simulink model "HVDCMMCInterconnection_O"  (R2023b)
settings: Solver=FixedStepDiscrete  StartTime=0.0  StopTime=10  RelTol=1e-3  EnableMultiTasking=on
PreLoadFcn:
  | HVDCMMCInterconnectionParam
StartFcn:
  | tic
StopFcn:
  | toc
values from neighbouring files (symbols this model uses):
  C_PM = 1.758e-3    (= 0.001758)    [HVDCMMCInterconnectionParam.m]
  Cfilter = 1/(Larm*wc2)    (= 4.78421193241e-05)    [HVDCMMCInterconnectionParam.m]
  Cg = 50e-9    (= 5e-08)    [HVDCMMCInterconnectionParam.m]
  Fc = Fnom*3.37    (= 168.5)    [HVDCMMCInterconnectionParam.m]
  Fnom = 50    [HVDCMMCInterconnectionParam.m]
  Ki_Ireg = 6    [HVDCMMCInterconnectionParam.m]
  Ki_Preg = 1.0    (= 1)    [HVDCMMCInterconnectionParam.m]
  Ki_Qreg = 1.0    (= 1)    [HVDCMMCInterconnectionParam.m]
  Ki_VDCreg = 100    [HVDCMMCInterconnectionParam.m]
  Kp_Ireg = 0.6    [HVDCMMCInterconnectionParam.m]
  Kp_Preg = 0.5/3    (= 0.166666666667)    [HVDCMMCInterconnectionParam.m]
  Kp_Qreg = 0.5/3    (= 0.166666666667)    [HVDCMMCInterconnectionParam.m]
  Kp_VDCreg = 4    [HVDCMMCInterconnectionParam.m]
  L_cable = 15e-3    (= 0.015)    [HVDCMMCInterconnectionParam.m]
  Larm = Larm_pu*(Zbase/(2*pi*Fnom))    (= 0.0529455974536)    [HVDCMMCInterconnectionParam.m]
  Lff = Larm_pu/2    (= 0.075)    [HVDCMMCInterconnectionParam.m]
  Limits_Ireg = [ 2.0  -2.0]    [HVDCMMCInterconnectionParam.m]
  Limits_Preg = [ 1.2, 0.8 ]    [HVDCMMCInterconnectionParam.m]
  Limits_Qreg = [ 0.25, -0.25 ]    [HVDCMMCInterconnectionParam.m]
  Limits_VDCreg = [ 2.0  -2.0]    [HVDCMMCInterconnectionParam.m]
  Lxfo = 0.12    [HVDCMMCInterconnectionParam.m]
  Nb_PM = 36    [HVDCMMCInterconnectionParam.m]
  Pnom = 1000e6    (= 1000000000)    [HVDCMMCInterconnectionParam.m]
  R_cable = 0.5    [HVDCMMCInterconnectionParam.m]
  R_startup = 400    [HVDCMMCInterconnectionParam.m]
  Rarm = Rarm_pu*Zbase    (= 0.1663335)    [HVDCMMCInterconnectionParam.m]
  Rff = Rarm_pu/2    (= 0.00075)    [HVDCMMCInterconnectionParam.m]
  Rfilter = 1/(Cfilter*w)*30    (= 1996.002)    [HVDCMMCInterconnectionParam.m]
  Rg = 100    [HVDCMMCInterconnectionParam.m]
  Rxfo = 0.003    [HVDCMMCInterconnectionParam.m]
  Slope_Pref = 0.5    [HVDCMMCInterconnectionParam.m]
  Slope_Qref = 0.5    [HVDCMMCInterconnectionParam.m]
  Slope_Vdc_ref = Vnom_dc/5    (= 128000)    [HVDCMMCInterconnectionParam.m]
  Tbrk1_On = 0.1    [HVDCMMCInterconnectionParam.m]
  Tbrk2_On = 1.0    (= 1)    [HVDCMMCInterconnectionParam.m]
  Tdeblock = 1.5    [HVDCMMCInterconnectionParam.m]
  Tfault = 9999    [HVDCMMCInterconnectionParam.m]
  Ton_Converter2 = 4    [HVDCMMCInterconnectionParam.m]
  Ton_PQreg = 4    [HVDCMMCInterconnectionParam.m]
  Ton_VDCreg = 1.5    [HVDCMMCInterconnectionParam.m]
  Ts = Ts_Control    (= 4e-05)    [HVDCMMCInterconnectionParam.m]
  Ts_Control = 40e-6    (= 4e-05)    [HVDCMMCInterconnectionParam.m]
  Ts_Power = 20e-6    (= 2e-05)    [HVDCMMCInterconnectionParam.m]
  Vnom_dc = 640e3    (= 640000)    [HVDCMMCInterconnectionParam.m]
  Vnom_prim = 400e3    (= 400000)    [HVDCMMCInterconnectionParam.m]
  Vnom_sec = 333e3    (= 333000)    [HVDCMMCInterconnectionParam.m]
undefined symbols (not defined in the file or in its folder): DiscIntNeverNeededParam, Pcc
libraries: spsSeriesRLCBranchLib x24, spsCurrentMeasurementLib x11, spsVoltageMeasurementLib x8, simulink x7, spsHalfBridgeMMCLib x6, powerlib_extras x3, spsIdealSwitchLib x3, spsBreakerLib x3, spsParallelRLCBranchLib x3, spsThreePhaseBreakerLib x2, spsMeanLib x2, spsSecondOrderFilterLib x2
(part 2 of 2)

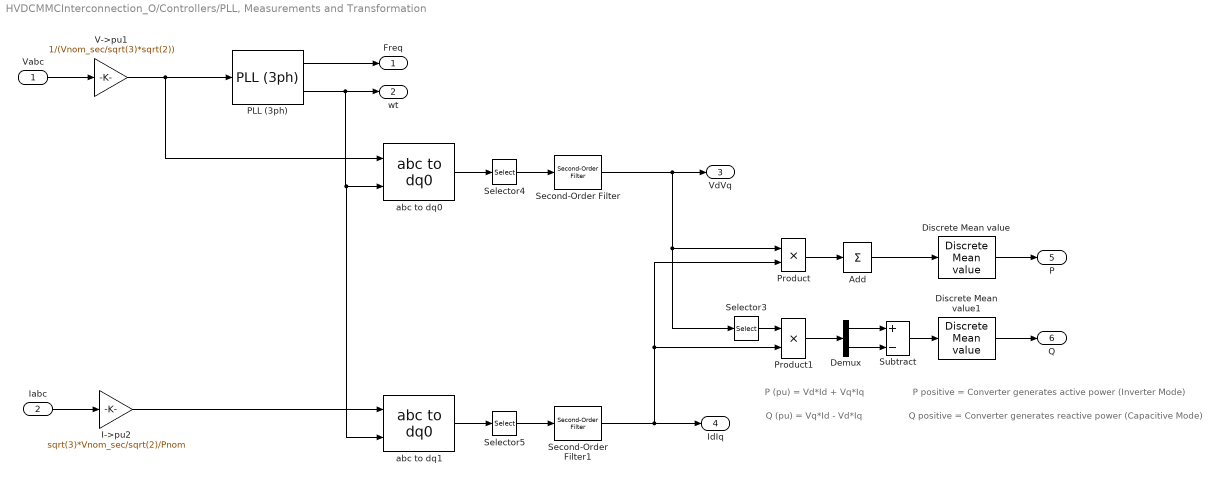
== system HVDCMMCInterconnection_O/Controllers/PLL, Measurements and Transformation ==
  note: P (pu) = Vd*Id + Vq*Iq
  note: Q (pu) = Vq*Id - Vd*Iq
  note: P positive = Converter generates active power (Inverter Mode)
  note: Q positive = Converter generates reactive power (Capacitive Mode)
  Vabc : Inport  PortDimensions=3
  Iabc : Inport  Port=2  PortDimensions=3
  Add : Sum  Inputs=1
  Demux : Demux  Outputs=2
  Discrete Mean value : powerlib_extras/Discrete Measurements/Discrete  Mean value  Freq=Fnom  Vinit=0  Ts=Ts
  Discrete Mean value1 : powerlib_extras/Discrete Measurements/Discrete  Mean value  Freq=Fnom  Vinit=0  Ts=Ts
  I->pu2 : Gain  Gain=sqrt(3)*Vnom_sec/sqrt(2)/Pnom  SaturateOnIntegerOverflow=on  OutDataTypeStr=Inherit: Same as input  ParamDataTypeStr=Inherit: Same as input
  PLL (3ph) : spsPLL3phLib/PLL (3ph)  Fmin=0.9*Fnom  Par_Init=[0, Fnom]  ParK=[180, 3200, 1]  TcD=1e-4  MaxRateChangeFreq=12  FilterCutOffFreq=25  Ts=Ts  AGC=on
  Product : Product  RndMeth=Zero
  Product1 : Product  RndMeth=Zero
  Second-Order Filter : spsSecondOrderFilterLib/Second-Order Filter  FilterType=Lowpass  Fo=Fn_filter  Zeta=Zeta_filter  Ts=Ts  Initialize=off  Vac_Init="[0,  0,  60]"  Vdc_Init=0  PlotResponse=off  FreqRange=[0, 500, 1]
  Second-Order Filter1 : spsSecondOrderFilterLib/Second-Order Filter  FilterType=Lowpass  Fo=Fn_filter  Zeta=Zeta_filter  Ts=Ts  Initialize=off  Vac_Init="[0,  0,  60]"  Vdc_Init=0  PlotResponse=off  FreqRange=[0, 500, 1]
  Selector3 : Selector  InputPortWidth=2  IndexOptions=Index vector (dialog)  Indices=[2 1]  OutputSizes=1
  Selector4 : Selector  InputPortWidth=3  IndexOptions=Index vector (dialog)  Indices=[1 2]  OutputSizes=1
  Selector5 : Selector  InputPortWidth=3  IndexOptions=Index vector (dialog)  Indices=[1 2]  OutputSizes=1
  Subtract : Sum  Inputs=+-
  V->pu1 : Gain  Gain=1/(Vnom_sec/sqrt(3)*sqrt(2))  SaturateOnIntegerOverflow=on  OutDataTypeStr=Inherit: Same as input  ParamDataTypeStr=Inherit: Same as input
  abc to dq0 : spsabctodq0Lib/abc to dq0  Alignment=90 degrees behind phase A axis
  abc to dq1 : spsabctodq0Lib/abc to dq0  Alignment=90 degrees behind phase A axis
  Freq : Outport
  wt : Outport  Port=2
  VdVq : Outport  Port=3
  IdIq : Outport  Port=4
  P : Outport  Port=5
  Q : Outport  Port=6
  wires:
  Selector3/1 -> Product1/1
  Discrete Mean value1/1 -> Q/1
  Discrete Mean value/1 -> P/1
  Second-Order Filter/1 -> VdVq/1, Product/1, Selector3/1
  Second-Order Filter1/1 -> IdIq/1, Product1/2, Product/2
  Product/1 -> Add/1
  Product1/1 -> Demux/1
  Demux/1 -> Subtract/1
  Demux/2 -> Subtract/2
  Add/1 -> Discrete Mean value/1
  Subtract/1 -> Discrete Mean value1/1
  abc to dq0/1 -> Selector4/1
  PLL (3ph)/1 -> Freq/1
  V->pu1/1 -> abc to dq0/1, PLL (3ph)/1
  Vabc/1 -> V->pu1/1
  PLL (3ph)/2 -> wt/1, abc to dq1/2, abc to dq0/2
  Iabc/1 -> I->pu2/1
  abc to dq1/1 -> Selector5/1
  I->pu2/1 -> abc to dq1/1
  Selector4/1 -> Second-Order Filter/1
  Selector5/1 -> Second-Order Filter1/1

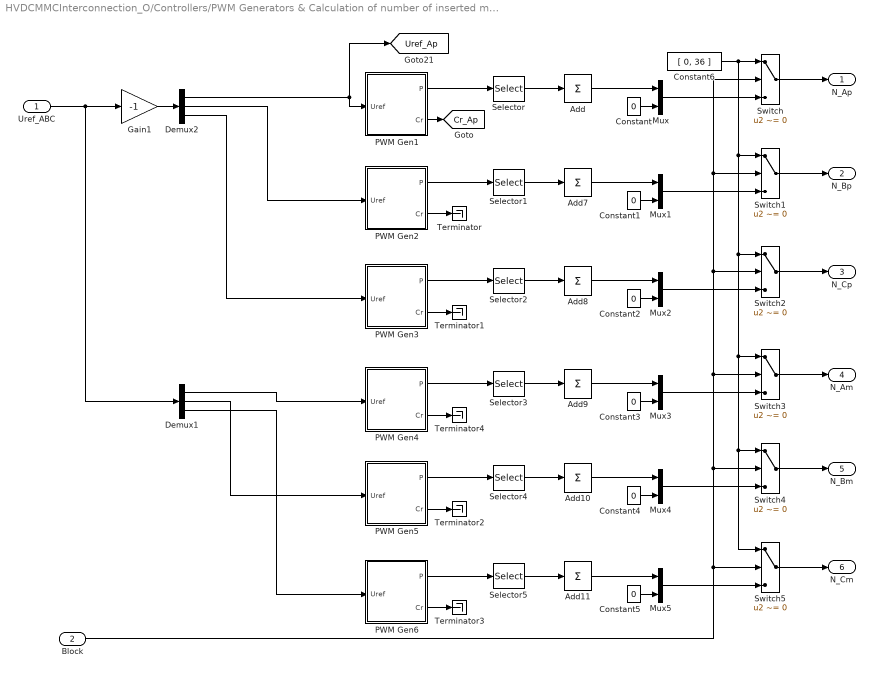
== system HVDCMMCInterconnection_O/Controllers/PWM Generators & Calculation of number of inserted modules (Nin) and number of blocked module (Nbl) ==
  Uref_ABC : Inport  PortDimensions=3
  Block : Inport  Port=2
  Add{,7..11} (6 alike) : Sum  Inputs=1
  Constant{,1..5} (6 alike) : Constant  Value=0
  Constant6 : Constant  Value=[ 0, 36 ]
  Demux1 : Demux  Outputs=3
  Demux2 : Demux  Outputs=3
  Gain1 : Gain  Gain=-1
  Mux{,1..5} (6 alike) : Mux  Inputs=2
  PWM Gen1 : Subsystem  mask(PWM generator for half-bridge MMC){n=Nb_PM, Fc=Fc, Ts=Ts_Power}
      mask prompts: n "Number of half-bridges"; Fc "Carriers frequency (Hz)"; Ts "Sample time (s)"
      mask init:
      | Tc=1/Fc;
      |         Pc= [ 0:360/n:360-360/n]*pi/180;
      |         Offset=Pc/(2*pi);
      |         Offset_Cr=Pc/(2*pi)*Tc;
      |         p=0;
      |         for m=1:2:2*n
      |             p=p+1;
      |             SelectPulsesPS(m)=p;
      |             SelectPulsesPS(m+1)=p+n;
      |         end
  PWM Gen2 : Subsystem  mask(PWM generator for half-bridge MMC){n=Nb_PM, Fc=Fc, Ts=Ts_Power}
      mask prompts: n "Number of half-bridges"; Fc "Carriers frequency (Hz)"; Ts "Sample time (s)"
      mask init: same as HVDCMMCInterconnection_O/Controllers/PWM Generators & Calculation of number of inserted modules (Nin) and number of blocked module (Nbl)/PWM Gen1
  PWM Gen3 : Subsystem  mask(PWM generator for half-bridge MMC){n=Nb_PM, Fc=Fc, Ts=Ts_Power}
      mask prompts: n "Number of half-bridges"; Fc "Carriers frequency (Hz)"; Ts "Sample time (s)"
      mask init: same as HVDCMMCInterconnection_O/Controllers/PWM Generators & Calculation of number of inserted modules (Nin) and number of blocked module (Nbl)/PWM Gen1
  PWM Gen4 : Subsystem  mask(PWM generator for half-bridge MMC){n=Nb_PM, Fc=Fc, Ts=Ts_Power}
      mask prompts: n "Number of half-bridges"; Fc "Carriers frequency (Hz)"; Ts "Sample time (s)"
      mask init: same as HVDCMMCInterconnection_O/Controllers/PWM Generators & Calculation of number of inserted modules (Nin) and number of blocked module (Nbl)/PWM Gen1
  PWM Gen5 : Subsystem  mask(PWM generator for half-bridge MMC){n=Nb_PM, Fc=Fc, Ts=Ts_Power}
      mask prompts: n "Number of half-bridges"; Fc "Carriers frequency (Hz)"; Ts "Sample time (s)"
      mask init: same as HVDCMMCInterconnection_O/Controllers/PWM Generators & Calculation of number of inserted modules (Nin) and number of blocked module (Nbl)/PWM Gen1
  PWM Gen6 : Subsystem  mask(PWM generator for half-bridge MMC){n=Nb_PM, Fc=Fc, Ts=Ts_Power}
      mask prompts: n "Number of half-bridges"; Fc "Carriers frequency (Hz)"; Ts "Sample time (s)"
      mask init: same as HVDCMMCInterconnection_O/Controllers/PWM Generators & Calculation of number of inserted modules (Nin) and number of blocked module (Nbl)/PWM Gen1
  Selector{,1..5} (6 alike) : Selector  InputPortWidth=72  IndexOptions=Index vector (dialog)  Indices=[1:2:71]  OutputSizes=1
  Switch{,1..5} (6 alike) : Switch  Criteria=u2 ~= 0  SaturateOnIntegerOverflow=off  InputSameDT=off
  Terminator{,1..4} (5 alike) : Terminator
  N_Ap : Outport
  N_Bp : Outport  Port=2
  N_Cp : Outport  Port=3
  N_Am : Outport  Port=4
  N_Bm : Outport  Port=5
  N_Cm : Outport  Port=6
  tag scope: Cr_Ap=global, Uref_Ap=global
  wires:
  PWM Gen4/2(Cr) -> Terminator4/1
  PWM Gen5/2(Cr) -> Terminator2/1
  Uref_ABC/1 -> Gain1/1, Demux1/1
  PWM Gen6/2(Cr) -> Terminator3/1
  PWM Gen2/2(Cr) -> Terminator/1
  Demux2/2 -> PWM Gen2/1(Uref)
  Demux2/1 -> PWM Gen1/1(Uref), [Uref_Ap]
  Gain1/1 -> Demux2/1
  PWM Gen1/2(Cr) -> [Cr_Ap]
  PWM Gen3/2(Cr) -> Terminator1/1
  Selector/1 -> Add/1
  Selector1/1 -> Add7/1
  Selector2/1 -> Add8/1
  Selector3/1 -> Add9/1
  Selector4/1 -> Add10/1
  Selector5/1 -> Add11/1
  Constant/1 -> Mux/2
  Add7/1 -> Mux1/1
  Constant1/1 -> Mux1/2
  Constant5/1 -> Mux5/2
  Switch/1 -> N_Ap/1
  Switch3/1 -> N_Am/1
  Mux1/1 -> Switch1/3
  Constant6/1 -> Switch/1, Switch5/1, Switch4/1, Switch3/1, Switch2/1, Switch1/1
  Constant2/1 -> Mux2/2
  Add9/1 -> Mux3/1
  Add8/1 -> Mux2/1
  Mux/1 -> Switch/3
  Switch1/1 -> N_Bp/1
  Constant4/1 -> Mux4/2
  Switch2/1 -> N_Cp/1
  Switch4/1 -> N_Bm/1
  Add/1 -> Mux/1
  Switch5/1 -> N_Cm/1
  Constant3/1 -> Mux3/2
  Add10/1 -> Mux4/1
  Add11/1 -> Mux5/1
  Block/1 -> Switch/2, Switch1/2, Switch2/2, Switch3/2, Switch4/2, Switch5/2
  Mux3/1 -> Switch3/3
  Mux4/1 -> Switch4/3
  Mux5/1 -> Switch5/3
  Mux2/1 -> Switch2/3
  PWM Gen6/1(P) -> Selector5/1
  PWM Gen5/1(P) -> Selector4/1
  PWM Gen4/1(P) -> Selector3/1
  PWM Gen3/1(P) -> Selector2/1
  PWM Gen2/1(P) -> Selector1/1
  PWM Gen1/1(P) -> Selector/1
  Demux2/3 -> PWM Gen3/1(Uref)
  Demux1/1 -> PWM Gen4/1(Uref)
  Demux1/3 -> PWM Gen6/1(Uref)
  Demux1/2 -> PWM Gen5/1(Uref)

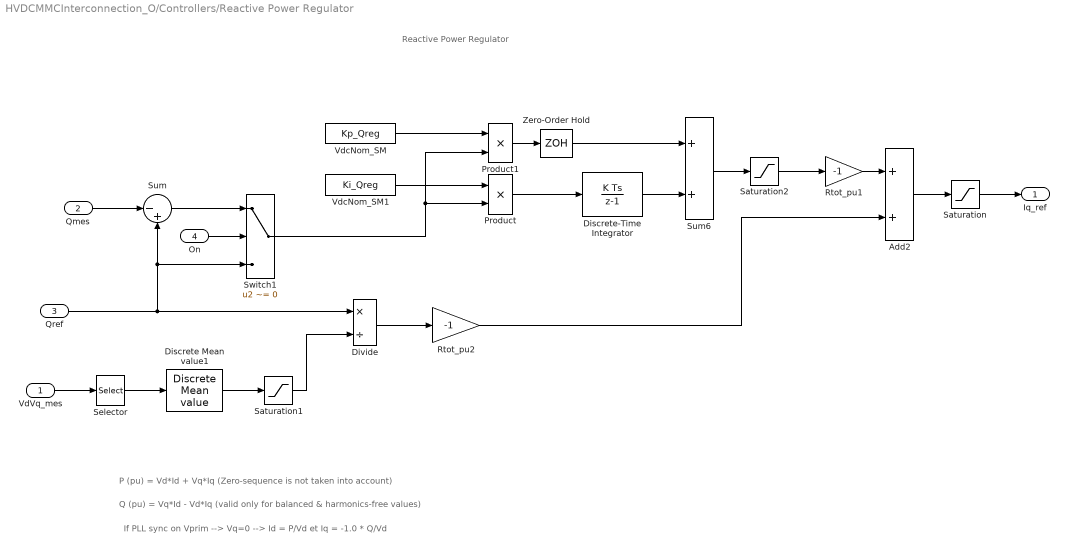
== system HVDCMMCInterconnection_O/Controllers/Reactive Power Regulator ==
  note: Reactive Power Regulator
  note: If PLL sync on Vprim --> Vq=0 --> Id = P/Vd et Iq = -1.0 * Q/Vd
  note: Q (pu) = Vq*Id - Vd*Iq (valid only for balanced & harmonics-free values)
  note: P (pu) = Vd*Id + Vq*Iq (Zero-sequence is not taken into account)
  VdVq_mes : Inport  PortDimensions=2
  Qmes : Inport  Port=2  PortDimensions=1
  Qref : Inport  Port=3  PortDimensions=1
  On : Inport  Port=4  PortDimensions=1
  Add2 : Sum
  Discrete Mean value1 : powerlib_extras/Discrete Measurements/Discrete  Mean value  Freq=Fnom  Vinit=0  Ts=Ts
  Discrete-Time Integrator : DiscreteIntegrator  SampleTime=Ts  LimitOutput=on  UpperSaturationLimit=Limits_Qreg(1)  LowerSaturationLimit=Limits_Qreg(2)  ICPrevOutput=DiscIntNeverNeededParam  ICPrevScaledInput=DiscIntNeverNeededParam
  Divide : Product  Inputs=*/
  Product : Product  RndMeth=Zero
  Product1 : Product  RndMeth=Zero
  Rtot_pu1 : Gain  Gain=-1  SaturateOnIntegerOverflow=on  OutDataTypeStr=Inherit: Same as input  ParamDataTypeStr=Inherit: Same as input
  Rtot_pu2 : Gain  Gain=-1  SaturateOnIntegerOverflow=on  OutDataTypeStr=Inherit: Same as input  ParamDataTypeStr=Inherit: Same as input
  Saturation : Saturate  UpperLimit=Limits_Qreg(1)  LowerLimit=Limits_Qreg(2)
  Saturation1 : Saturate  UpperLimit=2  LowerLimit=1e-6
  Saturation2 : Saturate  UpperLimit=Limits_Qreg(1)  LowerLimit=Limits_Qreg(2)
  Selector : Selector  InputPortWidth=2  IndexOptions=Index vector (dialog)  Indices=[1]  OutputSizes=1
  Sum : Sum  Inputs=|-+
  Sum6 : Sum  InputSameDT=on  SaturateOnIntegerOverflow=on  SampleTime=Ts  OutDataTypeStr=Inherit: Same as first input
  Switch1 : Switch  Criteria=u2 ~= 0  Threshold=0.5  OutDataTypeStr=double  SaturateOnIntegerOverflow=off  InputSameDT=off
  VdcNom_SM : Constant  Value=Kp_Qreg
  VdcNom_SM1 : Constant  Value=Ki_Qreg
  Zero-Order Hold : ZeroOrderHold  SampleTime=Ts
  Iq_ref : Outport
  wires:
  Saturation2/1 -> Rtot_pu1/1
  Saturation/1 -> Iq_ref/1
  Rtot_pu2/1 -> Add2/2
  Rtot_pu1/1 -> Add2/1
  Sum6/1 -> Saturation2/1
  Switch1/1 -> Product1/2, Product/2
  Sum/1 -> Switch1/1
  On/1 -> Switch1/2
  Add2/1 -> Saturation/1
  Product/1 -> Discrete-Time Integrator/1
  Product1/1 -> Zero-Order Hold/1
  VdcNom_SM/1 -> Product1/1
  VdcNom_SM1/1 -> Product/1
  Discrete-Time Integrator/1 -> Sum6/2
  Zero-Order Hold/1 -> Sum6/1
  Discrete Mean value1/1 -> Saturation1/1
  Saturation1/1 -> Divide/2
  Divide/1 -> Rtot_pu2/1
  Selector/1 -> Discrete Mean value1/1
  VdVq_mes/1 -> Selector/1
  Qmes/1 -> Sum/1
  Qref/1 -> Divide/1, Switch1/3, Sum/2

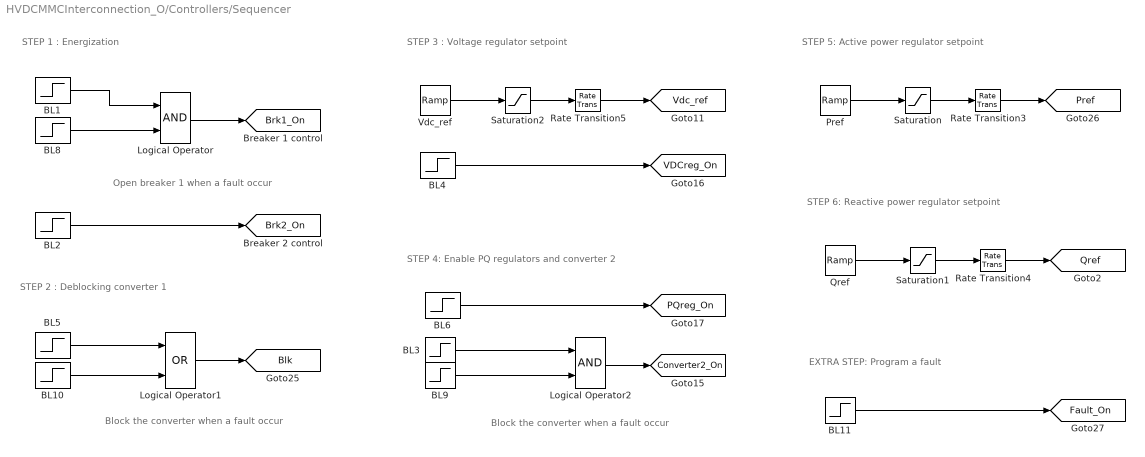
== system HVDCMMCInterconnection_O/Controllers/Sequencer ==
  note: Open breaker 1 when a fault occur
  note: Block the converter when a fault occur
  note: Block the converter when a fault occur
  note: STEP 6: Reactive power regulator setpoint
  note: STEP 4: Enable PQ regulators and converter 2
  note: STEP 5: Active power regulator setpoint
  note: STEP 3 : Voltage regulator setpoint
  note: STEP 2 : Deblocking converter 1
  note: STEP 1 : Energization
  note: EXTRA STEP: Program a fault
  BL1 : Step  Time=Tbrk1_On  SampleTime=Ts_Power
  BL10 : Step  Time=Tfault+Ts_Power  SampleTime=Ts_Power
  BL11 : Step  Time=Tfault  SampleTime=Ts_Power
  BL2 : Step  Time=Tbrk2_On  SampleTime=Ts_Power
  BL3 : Step  Time=Ton_Converter2  SampleTime=Ts_Power
  BL4 : Step  Time=Ton_VDCreg  SampleTime=Ts
  BL5 : Step  Time=Tdeblock  Before=1  After=0  SampleTime=Ts_Power
  BL6 : Step  Time=Ton_PQreg  SampleTime=Ts
  BL8 : Step  Time=Tfault + 1.95*(1/Fnom)  Before=1  After=0  SampleTime=Ts_Power
  BL9 : Step  Time=Tfault + 2*(1/Fnom)  Before=1  After=0  SampleTime=Ts_Power
  Logical Operator : Logic  AllPortsSameDT=off  OutDataTypeStr=boolean
  Logical Operator1 : Logic  Operator=OR  AllPortsSameDT=off  OutDataTypeStr=float('double')
  Logical Operator2 : Logic  AllPortsSameDT=off  OutDataTypeStr=boolean
  Pref : simulink/Sources/Ramp  slope=Slope_Pref  start=Tramping_Pref  InitialOutput=0
  Qref : simulink/Sources/Ramp  slope=Slope_Qref  start=Tramping_Qref  InitialOutput=0
  Rate Transition3 : RateTransition  OutPortSampleTime=Ts_Control
  Rate Transition4 : RateTransition  OutPortSampleTime=Ts_Control
  Rate Transition5 : RateTransition  OutPortSampleTime=Ts_Control
  Saturation : Saturate  UpperLimit=1  LowerLimit=-1
  Saturation1 : Saturate  UpperLimit=Limits_Qreg(1)  LowerLimit=Limits_Qreg(2)
  Saturation2 : Saturate  UpperLimit=Vnom_dc  LowerLimit=eps
  "Vdc_ref " : simulink/Sources/Ramp  slope=Slope_Vdc_ref  start=Tramping_Vdc_ref  InitialOutput=Vnom_sec*1.37
  tag scope: Blk=global, Brk1_On=global, Brk2_On=global, Converter2_On=global, Fault_On=global, PQreg_On=global, Pref=global, Qref=global, VDCreg_On=global, Vdc_ref=global
  wires:
  Saturation2/1 -> Rate Transition5/1
  Saturation1/1 -> Rate Transition4/1
  Pref/1 -> Saturation/1
  Qref/1 -> Saturation1/1
  Saturation/1 -> Rate Transition3/1
  Rate Transition3/1 -> [Pref]
  Rate Transition4/1 -> [Qref]
  Rate Transition5/1 -> [Vdc_ref]
  BL4/1 -> [VDCreg_On]
  BL6/1 -> [PQreg_On]
  "Vdc_ref "/1 -> Saturation2/1
  BL2/1 -> [Brk2_On]
  BL8/1 -> Logical Operator/2
  Logical Operator/1 -> [Brk1_On]
  BL1/1 -> Logical Operator/1
  BL9/1 -> Logical Operator2/2
  BL3/1 -> Logical Operator2/1
  Logical Operator2/1 -> [Converter2_On]
  Logical Operator1/1 -> [Blk]
  BL5/1 -> Logical Operator1/1
  BL10/1 -> Logical Operator1/2
  BL11/1 -> [Fault_On]

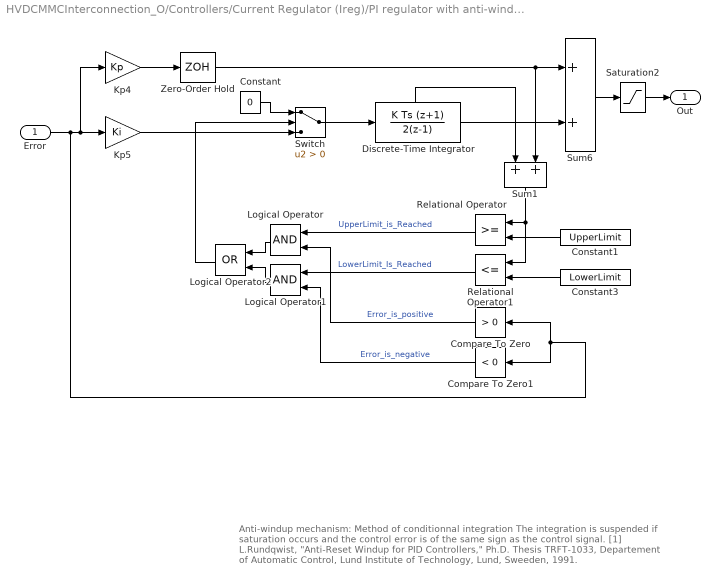
== system HVDCMMCInterconnection_O/Controllers/Current Regulator (Ireg)/PI regulator with anti-windup D ==
  note: Anti-windup mechanism: Method of conditionnal integration
      |
      | The integration is suspended if saturation occurs and the
      | control error is of the same sign as the control signal.
      |
      | [1] L.Rundqwist, "Anti-Reset Windup for PID Controllers," Ph.D. Thesis TRFT-1033,
      | Departement of Automatic Control, Lund Institute of Technology, Lund, Sweeden, 1991.
  Error : Inport  SampleTime=Ts
  Compare To Zero : simulink/Logic and Bit Operations/Compare To Zero  relop=>  OutDataTypeStr=uint8  ZeroCross=off
  Compare To Zero1 : simulink/Logic and Bit Operations/Compare To Zero  relop=<  OutDataTypeStr=uint8  ZeroCross=off
  Constant : Constant  Value=0
  Constant1 : Constant  Value=UpperLimit
  Constant3 : Constant  Value=LowerLimit
  Discrete-Time Integrator : DiscreteIntegrator  IntegratorMethod=Integration: Trapezoidal  InitialCondition=Init  SampleTime=Ts  LimitOutput=on  UpperSaturationLimit=UpperLimit  LowerSaturationLimit=LowerLimit  ShowStatePort=on  ICPrevOutput=DiscIntNeverNeededParam  ICPrevScaledInput=DiscIntNeverNeededParam
  Kp4 : Gain  Gain=Kp  SaturateOnIntegerOverflow=on  SampleTime=Ts  OutDataTypeStr=Inherit: Same as input  ParamDataTypeStr=Inherit: Same as input
  Kp5 : Gain  Gain=Ki  SaturateOnIntegerOverflow=on  SampleTime=Ts  OutDataTypeStr=Inherit: Same as input  ParamDataTypeStr=Inherit: Same as input
  Logical Operator : Logic  AllPortsSameDT=off  OutDataTypeStr=boolean
  Logical Operator1 : Logic  AllPortsSameDT=off  OutDataTypeStr=boolean
  Logical Operator2 : Logic  Operator=OR  AllPortsSameDT=off  OutDataTypeStr=boolean
  Relational Operator : RelationalOperator  OutDataTypeStr=boolean  InputSameDT=off
  Relational Operator1 : RelationalOperator  Operator=<=  OutDataTypeStr=boolean  InputSameDT=off
  Saturation2 : Saturate  UpperLimit=UpperLimit  LowerLimit=LowerLimit  SampleTime=Ts
  Sum1 : Sum  InputSameDT=on  SaturateOnIntegerOverflow=on  SampleTime=Ts  OutDataTypeStr=Inherit: Same as first input
  Sum6 : Sum  InputSameDT=on  SaturateOnIntegerOverflow=on  SampleTime=Ts  OutDataTypeStr=Inherit: Same as first input
  Switch : Switch  Criteria=u2 > Threshold  SaturateOnIntegerOverflow=off  InputSameDT=off
  Zero-Order Hold : ZeroOrderHold  SampleTime=Ts
  Out : Outport  SampleTime=Ts  InitialOutput=0
  wires:
  Constant/1 -> Switch/1
  Zero-Order Hold/1 -> Sum1/2, Sum6/1
  Discrete-Time Integrator/State -> Sum1/1
  Sum1/1 -> Relational Operator1/1, Relational Operator/1
  Logical Operator2/1 -> Switch/2
  Relational Operator/1 -> Logical Operator/1  "UpperLimit_is_Reached"
  Relational Operator1/1 -> Logical Operator1/1  "LowerLimit_Is_Reached"
  Constant1/1 -> Relational Operator/2
  Constant3/1 -> Relational Operator1/2
  Compare To Zero/1 -> Logical Operator/2  "Error_is_positive"
  Logical Operator/1 -> Logical Operator2/1
  Logical Operator1/1 -> Logical Operator2/2
  Compare To Zero1/1 -> Logical Operator1/2  "Error_is_negative"
  Error/1 -> Compare To Zero1/1, Compare To Zero/1, Kp4/1, Kp5/1
  Sum6/1 -> Saturation2/1
  Kp4/1 -> Zero-Order Hold/1
  Discrete-Time Integrator/1 -> Sum6/2
  Saturation2/1 -> Out/1
  Switch/1 -> Discrete-Time Integrator/1
  Kp5/1 -> Switch/3

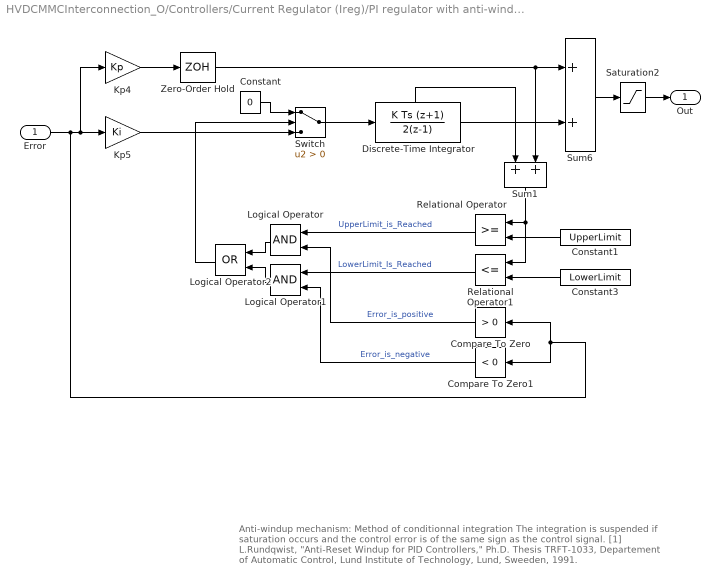
== system HVDCMMCInterconnection_O/Controllers/Current Regulator (Ireg)/PI regulator with anti-windup Q ==
  note: Anti-windup mechanism: Method of conditionnal integration
      |
      | The integration is suspended if saturation occurs and the
      | control error is of the same sign as the control signal.
      |
      | [1] L.Rundqwist, "Anti-Reset Windup for PID Controllers," Ph.D. Thesis TRFT-1033,
      | Departement of Automatic Control, Lund Institute of Technology, Lund, Sweeden, 1991.
  Error : Inport  SampleTime=Ts
  Compare To Zero : simulink/Logic and Bit Operations/Compare To Zero  relop=>  OutDataTypeStr=uint8  ZeroCross=off
  Compare To Zero1 : simulink/Logic and Bit Operations/Compare To Zero  relop=<  OutDataTypeStr=uint8  ZeroCross=off
  Constant : Constant  Value=0
  Constant1 : Constant  Value=UpperLimit
  Constant3 : Constant  Value=LowerLimit
  Discrete-Time Integrator : DiscreteIntegrator  IntegratorMethod=Integration: Trapezoidal  InitialCondition=Init  SampleTime=Ts  LimitOutput=on  UpperSaturationLimit=UpperLimit  LowerSaturationLimit=LowerLimit  ShowStatePort=on  ICPrevOutput=DiscIntNeverNeededParam  ICPrevScaledInput=DiscIntNeverNeededParam
  Kp4 : Gain  Gain=Kp  SaturateOnIntegerOverflow=on  SampleTime=Ts  OutDataTypeStr=Inherit: Same as input  ParamDataTypeStr=Inherit: Same as input
  Kp5 : Gain  Gain=Ki  SaturateOnIntegerOverflow=on  SampleTime=Ts  OutDataTypeStr=Inherit: Same as input  ParamDataTypeStr=Inherit: Same as input
  Logical Operator : Logic  AllPortsSameDT=off  OutDataTypeStr=boolean
  Logical Operator1 : Logic  AllPortsSameDT=off  OutDataTypeStr=boolean
  Logical Operator2 : Logic  Operator=OR  AllPortsSameDT=off  OutDataTypeStr=boolean
  Relational Operator : RelationalOperator  OutDataTypeStr=boolean  InputSameDT=off
  Relational Operator1 : RelationalOperator  Operator=<=  OutDataTypeStr=boolean  InputSameDT=off
  Saturation2 : Saturate  UpperLimit=UpperLimit  LowerLimit=LowerLimit  SampleTime=Ts
  Sum1 : Sum  InputSameDT=on  SaturateOnIntegerOverflow=on  SampleTime=Ts  OutDataTypeStr=Inherit: Same as first input
  Sum6 : Sum  InputSameDT=on  SaturateOnIntegerOverflow=on  SampleTime=Ts  OutDataTypeStr=Inherit: Same as first input
  Switch : Switch  Criteria=u2 > Threshold  SaturateOnIntegerOverflow=off  InputSameDT=off
  Zero-Order Hold : ZeroOrderHold  SampleTime=Ts
  Out : Outport  SampleTime=Ts  InitialOutput=0
  wires:
  Kp5/1 -> Switch/3
  Switch/1 -> Discrete-Time Integrator/1
  Saturation2/1 -> Out/1
  Discrete-Time Integrator/1 -> Sum6/2
  Kp4/1 -> Zero-Order Hold/1
  Sum6/1 -> Saturation2/1
  Error/1 -> Kp5/1, Kp4/1, Compare To Zero/1, Compare To Zero1/1
  Compare To Zero1/1 -> Logical Operator1/2  "Error_is_negative"
  Logical Operator1/1 -> Logical Operator2/2
  Logical Operator/1 -> Logical Operator2/1
  Compare To Zero/1 -> Logical Operator/2  "Error_is_positive"
  Constant3/1 -> Relational Operator1/2
  Constant1/1 -> Relational Operator/2
  Relational Operator1/1 -> Logical Operator1/1  "LowerLimit_Is_Reached"
  Relational Operator/1 -> Logical Operator/1  "UpperLimit_is_Reached"
  Logical Operator2/1 -> Switch/2
  Sum1/1 -> Relational Operator/1, Relational Operator1/1
  Discrete-Time Integrator/State -> Sum1/1
  Zero-Order Hold/1 -> Sum6/1, Sum1/2
  Constant/1 -> Switch/1

== system HVDCMMCInterconnection_O/Controllers/PWM Generators & Calculation of number of inserted modules (Nin) and number of blocked module (Nbl)/PWM Gen1 ==
  Uref : Inport
  Add6 : Sum
  Clock1 : DigitalClock  SampleTime=Ts
  Data Type Conversion : DataTypeConversion  OutDataTypeStr=double  SaturateOnIntegerOverflow=off  RndMeth=Floor
  Fc1 : Constant  Value=Tc
  Fc2 : Constant  Value=Fc
  Logical Operator2 : Logic  Operator=NOT  AllPortsSameDT=off  OutDataTypeStr=boolean
  Lookup Table1 : Lookup  InputValues=[0 .5 1]  Table=[-1 1 -1]  LookUpMeth=Interpolation-Use End Values  SaturateOnIntegerOverflow=off
  Math Function1 : Math  Operator=rem  SignedPower=on
  Mux6 : Mux  Inputs=2
  Phase_rad1 : Constant  Value=Offset_Cr
  Product2 : Product  RndMeth=Zero
  Relational Operator1 : RelationalOperator  OutDataTypeStr=boolean
  SelectPulses : Selector  InputPortWidth=2*n  IndexOptions=Index vector (dialog)  Indices=SelectPulsesPS  OutputSizes=1
  P : Outport
  Cr : Outport  Port=2
  wires:
  Data Type Conversion/1 -> P/1
  SelectPulses/1 -> Data Type Conversion/1
  Uref/1 -> Relational Operator1/1
  Lookup Table1/1 -> Relational Operator1/2, Cr/1
  Phase_rad1/1 -> Add6/2
  Fc2/1 -> Product2/2
  Logical Operator2/1 -> Mux6/2
  Mux6/1 -> SelectPulses/1
  Fc1/1 -> Math Function1/2
  Clock1/1 -> Add6/1
  Add6/1 -> Math Function1/1
  Product2/1 -> Lookup Table1/1
  Relational Operator1/1 -> Logical Operator2/1, Mux6/1
  Math Function1/1 -> Product2/1

== system HVDCMMCInterconnection_O/Controllers/PWM Generators & Calculation of number of inserted modules (Nin) and number of blocked module (Nbl)/PWM Gen2 ==
  Uref : Inport
  Add6 : Sum
  Clock1 : DigitalClock  SampleTime=Ts
  Data Type Conversion : DataTypeConversion  OutDataTypeStr=double  SaturateOnIntegerOverflow=off  RndMeth=Floor
  Fc1 : Constant  Value=Tc
  Fc2 : Constant  Value=Fc
  Logical Operator2 : Logic  Operator=NOT  AllPortsSameDT=off  OutDataTypeStr=boolean
  Lookup Table1 : Lookup  InputValues=[0 .5 1]  Table=[-1 1 -1]  LookUpMeth=Interpolation-Use End Values  SaturateOnIntegerOverflow=off
  Math Function1 : Math  Operator=rem  SignedPower=on
  Mux6 : Mux  Inputs=2
  Phase_rad1 : Constant  Value=Offset_Cr
  Product2 : Product  RndMeth=Zero
  Relational Operator1 : RelationalOperator  OutDataTypeStr=boolean
  SelectPulses : Selector  InputPortWidth=2*n  IndexOptions=Index vector (dialog)  Indices=SelectPulsesPS  OutputSizes=1
  P : Outport
  Cr : Outport  Port=2
  wires:
  Math Function1/1 -> Product2/1
  Relational Operator1/1 -> Mux6/1, Logical Operator2/1
  Product2/1 -> Lookup Table1/1
  Add6/1 -> Math Function1/1
  Clock1/1 -> Add6/1
  Fc1/1 -> Math Function1/2
  Mux6/1 -> SelectPulses/1
  Logical Operator2/1 -> Mux6/2
  Fc2/1 -> Product2/2
  Phase_rad1/1 -> Add6/2
  Lookup Table1/1 -> Cr/1, Relational Operator1/2
  Uref/1 -> Relational Operator1/1
  SelectPulses/1 -> Data Type Conversion/1
  Data Type Conversion/1 -> P/1

== system HVDCMMCInterconnection_O/Controllers/PWM Generators & Calculation of number of inserted modules (Nin) and number of blocked module (Nbl)/PWM Gen3 ==
  Uref : Inport
  Add6 : Sum
  Clock1 : DigitalClock  SampleTime=Ts
  Data Type Conversion : DataTypeConversion  OutDataTypeStr=double  SaturateOnIntegerOverflow=off  RndMeth=Floor
  Fc1 : Constant  Value=Tc
  Fc2 : Constant  Value=Fc
  Logical Operator2 : Logic  Operator=NOT  AllPortsSameDT=off  OutDataTypeStr=boolean
  Lookup Table1 : Lookup  InputValues=[0 .5 1]  Table=[-1 1 -1]  LookUpMeth=Interpolation-Use End Values  SaturateOnIntegerOverflow=off
  Math Function1 : Math  Operator=rem  SignedPower=on
  Mux6 : Mux  Inputs=2
  Phase_rad1 : Constant  Value=Offset_Cr
  Product2 : Product  RndMeth=Zero
  Relational Operator1 : RelationalOperator  OutDataTypeStr=boolean
  SelectPulses : Selector  InputPortWidth=2*n  IndexOptions=Index vector (dialog)  Indices=SelectPulsesPS  OutputSizes=1
  P : Outport
  Cr : Outport  Port=2
  wires:
  Data Type Conversion/1 -> P/1
  SelectPulses/1 -> Data Type Conversion/1
  Uref/1 -> Relational Operator1/1
  Lookup Table1/1 -> Relational Operator1/2, Cr/1
  Phase_rad1/1 -> Add6/2
  Fc2/1 -> Product2/2
  Logical Operator2/1 -> Mux6/2
  Mux6/1 -> SelectPulses/1
  Fc1/1 -> Math Function1/2
  Clock1/1 -> Add6/1
  Add6/1 -> Math Function1/1
  Product2/1 -> Lookup Table1/1
  Relational Operator1/1 -> Logical Operator2/1, Mux6/1
  Math Function1/1 -> Product2/1

== system HVDCMMCInterconnection_O/Controllers/PWM Generators & Calculation of number of inserted modules (Nin) and number of blocked module (Nbl)/PWM Gen4 ==
  Uref : Inport
  Add6 : Sum
  Clock1 : DigitalClock  SampleTime=Ts
  Data Type Conversion : DataTypeConversion  OutDataTypeStr=double  SaturateOnIntegerOverflow=off  RndMeth=Floor
  Fc1 : Constant  Value=Tc
  Fc2 : Constant  Value=Fc
  Logical Operator2 : Logic  Operator=NOT  AllPortsSameDT=off  OutDataTypeStr=boolean
  Lookup Table1 : Lookup  InputValues=[0 .5 1]  Table=[-1 1 -1]  LookUpMeth=Interpolation-Use End Values  SaturateOnIntegerOverflow=off
  Math Function1 : Math  Operator=rem  SignedPower=on
  Mux6 : Mux  Inputs=2
  Phase_rad1 : Constant  Value=Offset_Cr
  Product2 : Product  RndMeth=Zero
  Relational Operator1 : RelationalOperator  OutDataTypeStr=boolean
  SelectPulses : Selector  InputPortWidth=2*n  IndexOptions=Index vector (dialog)  Indices=SelectPulsesPS  OutputSizes=1
  P : Outport
  Cr : Outport  Port=2
  wires:
  Math Function1/1 -> Product2/1
  Relational Operator1/1 -> Mux6/1, Logical Operator2/1
  Product2/1 -> Lookup Table1/1
  Add6/1 -> Math Function1/1
  Clock1/1 -> Add6/1
  Fc1/1 -> Math Function1/2
  Mux6/1 -> SelectPulses/1
  Logical Operator2/1 -> Mux6/2
  Fc2/1 -> Product2/2
  Phase_rad1/1 -> Add6/2
  Lookup Table1/1 -> Cr/1, Relational Operator1/2
  Uref/1 -> Relational Operator1/1
  SelectPulses/1 -> Data Type Conversion/1
  Data Type Conversion/1 -> P/1

== system HVDCMMCInterconnection_O/Controllers/PWM Generators & Calculation of number of inserted modules (Nin) and number of blocked module (Nbl)/PWM Gen5 ==
  Uref : Inport
  Add6 : Sum
  Clock1 : DigitalClock  SampleTime=Ts
  Data Type Conversion : DataTypeConversion  OutDataTypeStr=double  SaturateOnIntegerOverflow=off  RndMeth=Floor
  Fc1 : Constant  Value=Tc
  Fc2 : Constant  Value=Fc
  Logical Operator2 : Logic  Operator=NOT  AllPortsSameDT=off  OutDataTypeStr=boolean
  Lookup Table1 : Lookup  InputValues=[0 .5 1]  Table=[-1 1 -1]  LookUpMeth=Interpolation-Use End Values  SaturateOnIntegerOverflow=off
  Math Function1 : Math  Operator=rem  SignedPower=on
  Mux6 : Mux  Inputs=2
  Phase_rad1 : Constant  Value=Offset_Cr
  Product2 : Product  RndMeth=Zero
  Relational Operator1 : RelationalOperator  OutDataTypeStr=boolean
  SelectPulses : Selector  InputPortWidth=2*n  IndexOptions=Index vector (dialog)  Indices=SelectPulsesPS  OutputSizes=1
  P : Outport
  Cr : Outport  Port=2
  wires:
  Data Type Conversion/1 -> P/1
  SelectPulses/1 -> Data Type Conversion/1
  Uref/1 -> Relational Operator1/1
  Lookup Table1/1 -> Relational Operator1/2, Cr/1
  Phase_rad1/1 -> Add6/2
  Fc2/1 -> Product2/2
  Logical Operator2/1 -> Mux6/2
  Mux6/1 -> SelectPulses/1
  Fc1/1 -> Math Function1/2
  Clock1/1 -> Add6/1
  Add6/1 -> Math Function1/1
  Product2/1 -> Lookup Table1/1
  Relational Operator1/1 -> Logical Operator2/1, Mux6/1
  Math Function1/1 -> Product2/1

== system HVDCMMCInterconnection_O/Controllers/PWM Generators & Calculation of number of inserted modules (Nin) and number of blocked module (Nbl)/PWM Gen6 ==
  Uref : Inport
  Add6 : Sum
  Clock1 : DigitalClock  SampleTime=Ts
  Data Type Conversion : DataTypeConversion  OutDataTypeStr=double  SaturateOnIntegerOverflow=off  RndMeth=Floor
  Fc1 : Constant  Value=Tc
  Fc2 : Constant  Value=Fc
  Logical Operator2 : Logic  Operator=NOT  AllPortsSameDT=off  OutDataTypeStr=boolean
  Lookup Table1 : Lookup  InputValues=[0 .5 1]  Table=[-1 1 -1]  LookUpMeth=Interpolation-Use End Values  SaturateOnIntegerOverflow=off
  Math Function1 : Math  Operator=rem  SignedPower=on
  Mux6 : Mux  Inputs=2
  Phase_rad1 : Constant  Value=Offset_Cr
  Product2 : Product  RndMeth=Zero
  Relational Operator1 : RelationalOperator  OutDataTypeStr=boolean
  SelectPulses : Selector  InputPortWidth=2*n  IndexOptions=Index vector (dialog)  Indices=SelectPulsesPS  OutputSizes=1
  P : Outport
  Cr : Outport  Port=2
  wires:
  Math Function1/1 -> Product2/1
  Relational Operator1/1 -> Mux6/1, Logical Operator2/1
  Product2/1 -> Lookup Table1/1
  Add6/1 -> Math Function1/1
  Clock1/1 -> Add6/1
  Fc1/1 -> Math Function1/2
  Mux6/1 -> SelectPulses/1
  Logical Operator2/1 -> Mux6/2
  Fc2/1 -> Product2/2
  Phase_rad1/1 -> Add6/2
  Lookup Table1/1 -> Cr/1, Relational Operator1/2
  Uref/1 -> Relational Operator1/1
  SelectPulses/1 -> Data Type Conversion/1
  Data Type Conversion/1 -> P/1
